simulink model "ass1"  (R2019a)
settings: Solver=FixedStepDiscrete  StartTime=0.0  StopTime=10.0  RelTol=1e-3
settings Model: Creator=ajayp  LastModifiedBy=ajayp

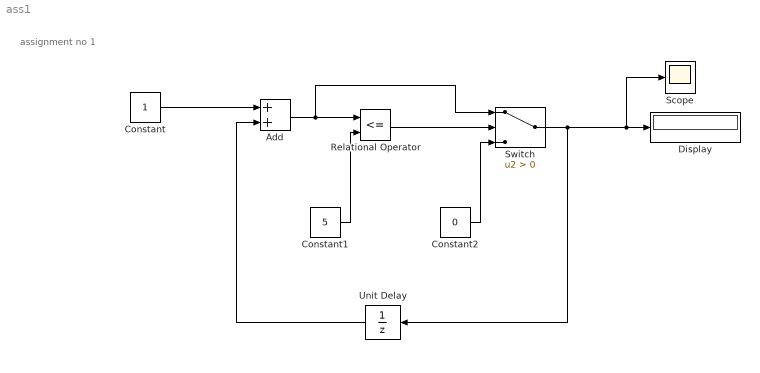
== system ass1 ==
  note: assignment no 1
  Add : Sum
  Constant : Constant
  Constant1 : Constant  Value=5
  Constant2 : Constant  Value=0
  Display : Display
  Relational Operator : RelationalOperator  Operator=<=  OutDataTypeStr=boolean  RndMeth=Simplest
  Scope : Scope
  Switch : Switch  Criteria=u2 > Threshold
  Unit Delay : UnitDelay  InitialCondition=-1  SampleTime=-1  HasFrameUpgradeWarning=on
  wires:
  Switch/1 -> Unit Delay/1, Scope/1, Display/1
  Relational Operator/1 -> Switch/2
  Add/1 -> Switch/1, Relational Operator/1
  Constant/1 -> Add/1
  Constant2/1 -> Switch/3
  Constant1/1 -> Relational Operator/2
  Unit Delay/1 -> Add/2
